simulink model "das2test"  (Simulink 8.8)
settings: Solver=ode4  StartTime=0.0  StopTime=10  FixedStep=Auto  RelTol=1e-3  EnableMultiTasking=on
PostLoadFcn:
  | , if any(exist('dsrtsu_mdlpostloadfcn', 'file') == [2, 3, 6]), try dsrtsu_mdlpostloadfcn('Execute', bdroot); catch fprintf('Error in PostLoadFcn (dsrtsu_mdlpostloadfcn) for model "%s":\n %s\n', bdroot, lasterr); end, end,
libraries: simulink x1
PreSaveFcn:
  | , if any(exist('dsmpb_private', 'file') == [2, 3, 6]), try, dsmpb_private('dsmpb_mdlclblib', 'PreSave', bdroot); catch, disp(lasterr); end, end,
CloseFcn:
  | , if any(exist('dsmpb_private', 'file') == [2, 3, 6]), try, dsmpb_private('dsmpb_mdlclblib', 'Close', bdroot); catch, disp(lasterr); end, end,
settings Model: DSMPB_DATASERVER_ModelPortLibVersion1=8  DSMPB_DATASERVER_DataServerVersion1=6  DSMPB_DATASERVER_DataServerStreamVersion1=3  Creator=chadwick  LastModifiedBy=labuser  ParamWorkspaceSource=ReferencedWorkspace  ExtModeAutoUpdateStatusClock=off
settings SolverCC: EnableConcurrentExecution=on
settings DataIOCC: MaxDataPoints=20000  SaveFinalState=on  SaveOutput=off  SignalLogging=off  SaveTime=off
settings OptimizationCC: BlockReduction=off  DefaultParameterBehavior=Inlined  OptimizeBlockIOStorage=off  BufferReuse=off  GlobalBufferReuse=off  ExpressionFolding=off  ExpressionDepthLimit=2147483647  LocalBlockOutputs=off  InitFltsAndDblsToZero=on  LifeSpan=auto
settings DebuggingCC: SaveWithParameterizedLinksMsg=none  SignalResolutionControl=TryResolveAllWithWarning  SolverPrmCheckMsg=warning  MultiTaskDSMMsg=warning  MultiTaskCondExecSysMsg=none  StrictBusMsg=Warning
settings HardwareCC: ProdIntDivRoundTo=Zero  ProdEndianess=LittleEndian  ProdLongLongMode=on  ProdHWDeviceType=Generic->32-bit x86 compatible
settings ModelReferenceCC: ModelReferenceNumInstancesAllowed=Single
settings SFSimCC: SimParseCustomCode=off
settings RTWCC: SystemTargetFile=slrt.tlc  TemplateMakefile=slrt_default_tmf  Description=Simulink Real-Time  CustomInclude=..\..\..\tools\sdbio\trunk\ ..\..\..\das2\model\trunk\ ..\..\..\das2\das2sim\trunk\  CustomSource=sdbio.c sdlib.c model_d.c
settings SimulinkRealTimeCC: TargetFcnLib=ansi_tfl_tmw.mat  RL32ModeModifier=Freerun  RL32LogBufSizeModifier=20000

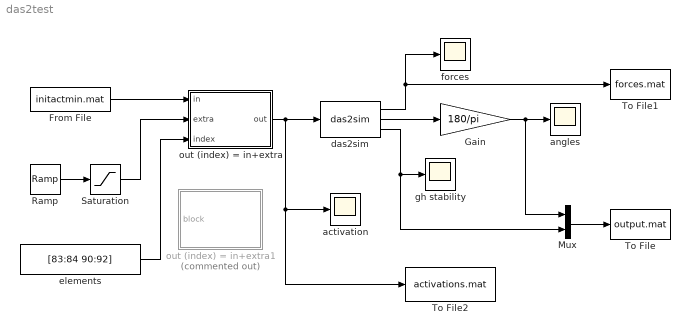
== system das2test ==
  From File : FromFile  FileName=initactmin.mat  SampleTime=0.001
  Gain : Gain  Gain=180/pi
  Mux : Mux  Inputs=2
  Ramp : simulink/Sources/Ramp  slope=0.2  start=1  X0=0
  Saturation : Saturate  UpperLimit=1  LowerLimit=0
  To File : ToFile  Filename=output.mat  MatrixName=output
      settings: Decimation=10
  To File1 : ToFile  Filename=forces.mat  MatrixName=forces
      settings: Decimation=10
  To File2 : ToFile  Filename=activations.mat  MatrixName=act
      settings: Decimation=20
  activation : Scope
  angles : Scope
  das2sim : S-Function  FunctionName=das2sim  SFunctionDeploymentMode=off  EnableBusSupport=off
  elements : Constant  Value=[83:84 90:92]
  forces : Scope
  gh stability : Scope
  out (index) = in+extra : MATLAB Function  TreatAsAtomicUnit=on
  out (index) = in+extra1 : MATLAB Function  Commented=on  TreatAsAtomicUnit=on
  wires:
  das2sim/2 -> Gain/1
  Gain/1 -> angles/1, Mux/1
  das2sim/3 -> gh stability/1, Mux/2
  out (index) = in+extra/1(out) -> das2sim/1, activation/1, To File2/1
  Mux/1 -> To File/1
  das2sim/1 -> forces/1, To File1/1
  From File/1 -> out (index) = in+extra/1(in)
  Ramp/1 -> Saturation/1
  elements/1 -> out (index) = in+extra/3(index)
  Saturation/1 -> out (index) = in+extra/2(extra)

== matlab function out (index) = in+extra1 ==
  data: block input double
function injection(block)
%   injection: M-file S-function that adds a signal (input 2) to specified elements
%   of the input vector (input 1)
%   the elements are specified in the parameters dialog
%
%   Dimitra Blana - September 11th 2007

setup(block);

%endfunction

%% S-function methods

function setup(block)

% Register number of ports
block.NumInputPorts  = 2;
block.NumOutputPorts = 1;
block.NumDialogPrms     = 1;
block.DialogPrmsTunable = {'Nontunable'};

% Setup port properties to be inherited or dynamic
block.SetPreCompInpPortInfoToDynamic;
block.SetPreCompOutPortInfoToDynamic;

block.InputPort(1).DatatypeID  = 0;  % double
block.InputPort(1).Complexity  = 'Real';
block.InputPort(1).Dimensions = 102;

block.InputPort(2).DatatypeID  = 0;  % double
block.InputPort(2).Complexity  = 'Real';
block.InputPort(2).Dimensions = 1;
  
block.OutputPort(1).DatatypeID  = 0; % double
block.OutputPort(1).Complexity  = 'Real';
block.OutputPort(1).Dimensions = 102;

block.SampleTimes = [-1 0];

block.RegBlockMethod('Outputs', @Outputs);

block.SetAccelRunOnTLC(false);

%endfunction
function Outputs(block)

input_act = block.InputPort(1).Data;
extra_act = block.InputPort(2).Data;
index = block.DialogPrm(1).Data;

new_act = input_act;
for i=index
    new_act(i)=input_act(i)+extra_act;
end

block.OutputPort(1).Data = new_act;

%endfunction

== matlab function out (index) = in+extra ==
  data: in input double; out output double; extra input double; index input double
function out = inject(in,extra,index)
% adds an EXTRA signal to specified elements (INDEX) of the IN vector

out = in;
for i=index
    out(i)=in(i)+extra;
end
